simulink model "simulink_st"  (R2025a)
settings: Solver=VariableStepAuto  StartTime=0.0  StopTime=10.0  RelTol=1e-3
settings Model: Creator=nischal  LastModifiedBy=nischal

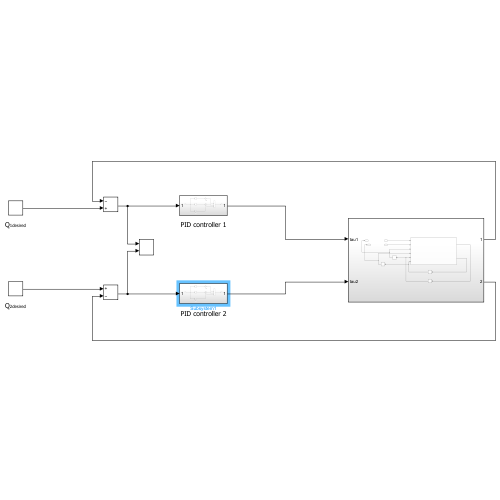
[thumbnail: Simulink's stored preview of the top-level diagram]
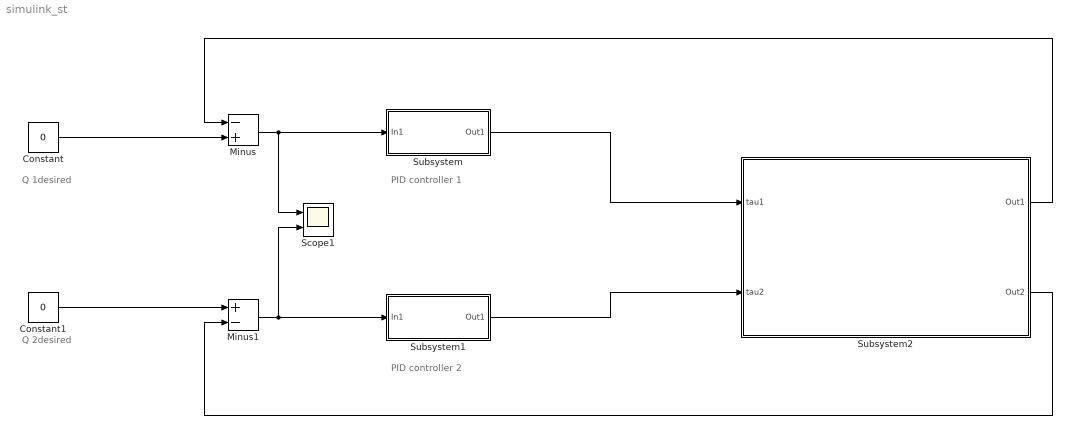
== system simulink_st ==
  note: Q 1desired
  note: PID controller 1
  note: PID controller 2
  note: Q 2desired
  Constant : Constant  Value=0
  Constant1 : Constant  Value=0
  Minus : Sum  Inputs=-+
  Minus1 : Sum  Inputs=+-
  Scope1 : Scope  NumInputPorts=2
      settings: ActiveDisplayYMinimum=-0.22730611378546087  ActiveDisplayYMaximum=0.045565535424076112
  Subsystem : Subsystem
  Subsystem1 : Subsystem
  Subsystem2 : Subsystem
  wires:
  Minus1/1 -> Scope1/2, Subsystem1/1(In1)
  Minus/1 -> Scope1/1, Subsystem/1(In1)
  Constant1/1 -> Minus1/1
  Subsystem/1(Out1) -> Subsystem2/1(tau1)
  Subsystem1/1(Out1) -> Subsystem2/2(tau2)
  Constant/1 -> Minus/2
  Subsystem2/2(Out2) -> Minus1/2
  Subsystem2/1(Out1) -> Minus/1

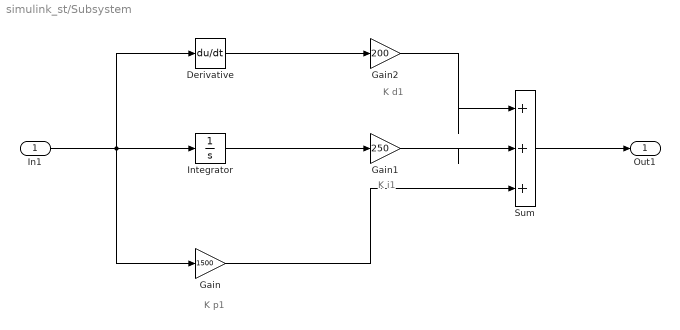
== system simulink_st/Subsystem ==
  note: K d1
  note: K i1
  note: K p1
  In1 : Inport
  Derivative : Derivative
  Gain : Gain  Gain=1500
  Gain1 : Gain  Gain=250
  Gain2 : Gain  Gain=200
  Integrator : Integrator
  Sum : Sum  Inputs=|+++
  Out1 : Outport
  wires:
  In1/1 -> Gain/1, Derivative/1, Integrator/1
  Integrator/1 -> Gain1/1
  Derivative/1 -> Gain2/1
  Gain2/1 -> Sum/1
  Gain1/1 -> Sum/2
  Gain/1 -> Sum/3
  Sum/1 -> Out1/1

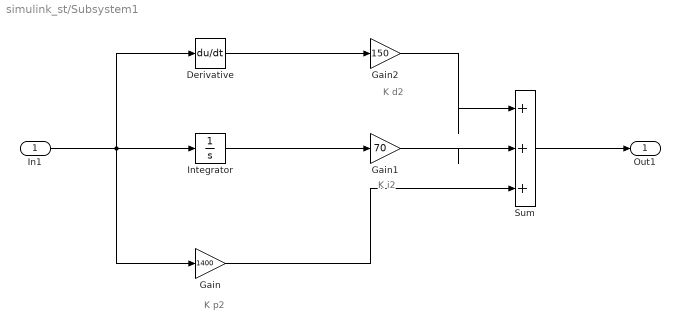
== system simulink_st/Subsystem1 ==
  note: K d2
  note: K i2
  note: K p2
  In1 : Inport
  Derivative : Derivative
  Gain : Gain  Gain=1400
  Gain1 : Gain  Gain=70
  Gain2 : Gain  Gain=150
  Integrator : Integrator
  Sum : Sum  Inputs=|+++
  Out1 : Outport
  wires:
  In1/1 -> Gain/1, Derivative/1, Integrator/1
  Integrator/1 -> Gain1/1
  Derivative/1 -> Gain2/1
  Gain2/1 -> Sum/1
  Gain1/1 -> Sum/2
  Gain/1 -> Sum/3
  Sum/1 -> Out1/1

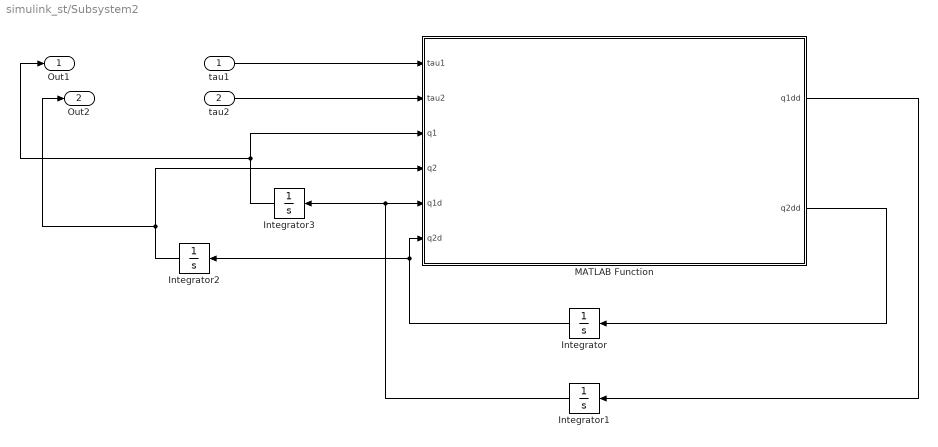
== system simulink_st/Subsystem2 ==
  tau1 : Inport
  tau2 : Inport  Port=2
  Integrator : Integrator
  Integrator1 : Integrator
  Integrator2 : Integrator  InitialCondition=0.15
  Integrator3 : Integrator  InitialCondition=0.2
  MATLAB Function : MATLAB Function  TreatAsAtomicUnit=on
  Out1 : Outport
  Out2 : Outport  Port=2
  wires:
  tau2/1 -> MATLAB Function/2(tau2)
  tau1/1 -> MATLAB Function/1(tau1)
  MATLAB Function/2(q2dd) -> Integrator/1
  MATLAB Function/1(q1dd) -> Integrator1/1
  Integrator/1 -> MATLAB Function/6(q2d), Integrator2/1
  Integrator1/1 -> Integrator3/1, MATLAB Function/5(q1d)
  Integrator3/1 -> MATLAB Function/3(q1), Out1/1
  Integrator2/1 -> Out2/1, MATLAB Function/4(q2)

== matlab function simulink_st/Subsystem2/MATLAB Function ==
  data: tau1 input; q1dd output; tau2 input; q2dd output; q1 input; q2 input; q1d input; q2d input
function [q1dd, q2dd] = manipulator_dynamics(tau1, tau2, q1, q2, q1d, q2d)
% This function calculates the forward dynamics of a 2-link planar
% manipulator.
%
% Inputs:
%   tau1, tau2: Joint torques for link 1 and link 2
%   q1, q2:     Joint angles for link 1 and link 2
%   q1d, q2d:   Joint velocities for link 1 and link 2
%
% Outputs:
%   q1dd, q2dd: Joint accelerations for link 1 and link 2

% Define system parameters. 
% Using 'persistent' is more efficient as they are only initialized once.
persistent m1 m2 l1 l2 g;
if isempty(m1)
    m1 = 5;     % kg
    m2 = 3;     % kg
    l1 = 0.25;  % m
    l2 = 0.15;  % m
    g = 9.81;   % m/s^2
end

% For easier matrix calculations, group inputs into vectors
tau = [tau1; tau2];
q_d = [q1d; q2d];

% --- Calculate the Inertia Matrix M(q) ---
% M = [M11, M12; M21, M22]
M11 = (m1 + m2)*l1^2 + m2*l2^2 + 2*m2*l1*l2*cos(q2);
M12 = m2*l2^2 + m2*l1*l2*cos(q2);
M21 = m2*l2^2 + m2*l1*l2*cos(q2);
M22 = m2*l2^2;

M = [M11, M12; 
     M21, M22];

% --- Calculate the Coriolis and Centrifugal Matrix C(q, q_d) ---
% C = [C11, C12; C21, C22]
h = -m2*l1*l2*sin(q2);

C11 = h * q2d;
C12 = h * (q1d + q2d);
C21 = -h * q1d;
C22 = 0;

C = [C11, C12; 
     C21, C22];

% --- Calculate the Gravity Vector G(q) ---
% G = [G1; G2]
G1 = (m1+m2)*g*l1*cos(q1) + m2*g*l2*cos(q1+q2);
G2 = m2*g*l2*cos(q1+q2);

G = [G1; G2];

% --- Solve the Dynamic Equation for Joint Accelerations ---
% The dynamic equation is: M(q)*q_dd + C(q,q_d)*q_d + G(q) = tau
% We rearrange it to solve for q_dd: q_dd = inv(M) * (tau - C*q_d - G)
% Using the backslash operator '\' is more numerically stable and
% efficient in MATLAB than using inv(M).

q_dd = M \ (tau - C*q_d - G);

% Assign the calculated accelerations to the output variables
q1dd = q_dd(1);
q2dd = q_dd(2);

end
